simulink model "sampleModel1845"  (R2023a)
settings: Solver=VariableStepAuto  StartTime=0.0  StopTime=10.0  RelTol=1e-3
libraries: simulink x4, hdlsllib x2
settings Model: Creator=user1  LastModifiedBy=user1

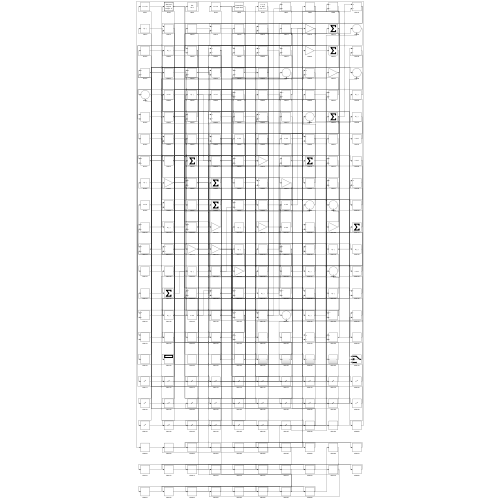
[thumbnail: Simulink's stored preview of the top-level diagram]
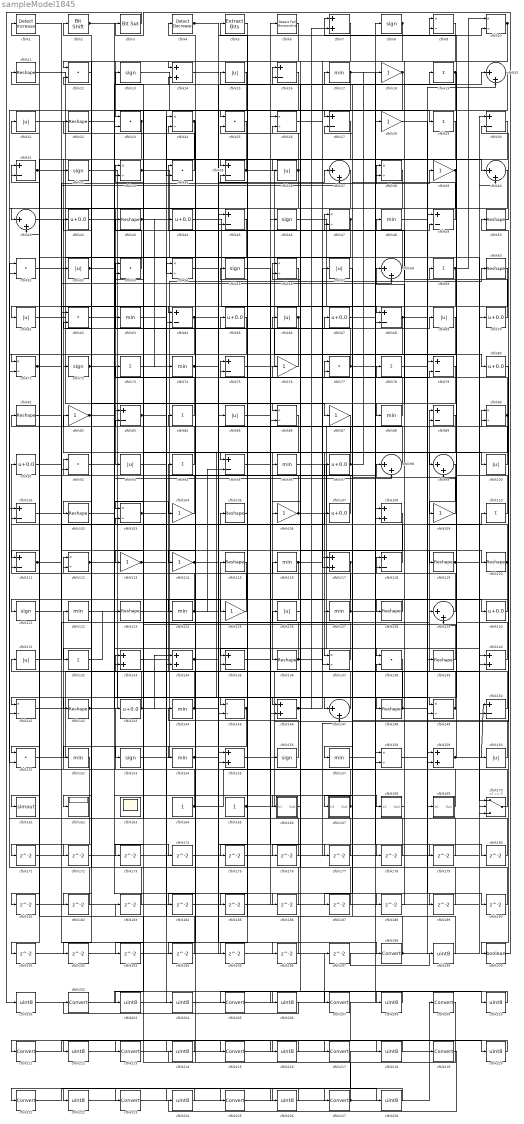
== system sampleModel1845 ==
  cfblk1 : simulink/Logic and Bit Operations/Detect Increase  vinit=0.0  OutDataTypeStr=boolean
      settings: LibrarySourceBlock=|
      | hdlsllib/Logic and Bit
      | Operations/Detect
      | Increase
  cfblk{9..10,24,26,33,38,47,54,56,71,86,90,103,112,137,141,145,149,158} (19 alike) : Product  Inputs=*/  RndMeth=Zero  SaturateOnIntegerOverflow=on
  cfblk{15,21,36,52,57,61,66,69,85,93,100,126,131,160} (14 alike) : Abs  SaturateOnIntegerOverflow=off
  cfblk{16,27,30..31,35,45,49,64,68,75,79,83,89,95,101,111,118,135,150} (19 alike) : Sum  Inputs=+-
  cfblk{11,22,43,50,60,81,102,105,115,119..120,123,128,136,139,142,148} (17 alike) : Reshape
  cfblk{18,28,39,76,82,87,104,106,109,113..114,125} (12 alike) : Gain
  cfblk{42,44,65,67,70,80,91,97,107,130,143} (11 alike) : Bias  Bias=0.0  SaturateOnIntegerOverflow=off
  cfblk{7,14,108,117,133..134,140,146,155,159} (10 alike) : Sum
  cfblk{19,29,59,73,78,84,94,110,132} (9 alike) : Sum  Inputs=+
  cfblk{17,48,63,74,88,96,116,122,124,127,144,152,154,157} (14 alike) : MinMax
  cfblk{12,23,25,34,51,53,62,77,92,138,151} (11 alike) : DotProduct  OutDataTypeStr=Inherit: Inherit via internal rule
  cfblk{8,13,32,46,55,72,121,153,156} (9 alike) : Signum
  cfblk{20,37,40..41,58,98..99,129,147} (9 alike) : Sum  Inputs=|++
  cfblk161 : ToWorkspace  VariableName=simout  SaveFormat=Timeseries  SampleTime=-1
  cfblk162 : Display
  cfblk163 : Scope
      settings: Floating=on
  cfblk164 : Constant  SampleTime=-1
  cfblk165 : Constant  SampleTime=-1
  cfblk166 : Subsystem
      settings: LibrarySourceBlock=|
      | hdlsllib/Ports &
      | Subsystems/Subsystem
  cfblk167 : Subsystem
      settings: LibrarySourceBlock=|
      | hdlsllib/Ports &
      | Subsystems/Subsystem
  cfblk168 : Subsystem
      settings: LibrarySourceBlock=|
      | hdlsllib/Ports &
      | Subsystems/Subsystem
  cfblk169 : Subsystem
      settings: LibrarySourceBlock=|
      | hdlsllib/Ports &
      | Subsystems/Subsystem
  cfblk170 : Switch  SaturateOnIntegerOverflow=off  InputSameDT=off
  cfblk{171..197} (27 alike) : Delay  SampleTime=1
  cfblk{198,202,205,207,209,211,213,215,217,219,221,223,225,227} (14 alike) : DataTypeConversion  SaturateOnIntegerOverflow=off  RndMeth=Floor
  cfblk{199,201,203..204,206,208,210,212,214,216,218,220,222,224,226,228} (16 alike) : DataTypeConversion  OutDataTypeStr=uint8  SaturateOnIntegerOverflow=off  RndMeth=Floor
  cfblk2 : hdlsllib/Logic and Bit Operations/Bit Shift  mode=Shift Left Logical  N=0
  cfblk200 : DataTypeConversion  OutDataTypeStr=boolean  SaturateOnIntegerOverflow=off  RndMeth=Floor
  cfblk3 : simulink/Logic and Bit Operations/Bit Set  iBit=0
      settings: LibrarySourceBlock=|
      | hdlsllib/Logic and Bit
      | Operations/Bit Set
  cfblk4 : simulink/Logic and Bit Operations/Detect Decrease  vinit=0.0  OutDataTypeStr=boolean
      settings: LibrarySourceBlock=|
      | hdlsllib/Logic and Bit
      | Operations/Detect
      | Decrease
  cfblk5 : simulink/Logic and Bit Operations/Extract Bits  bitsToExtract=Upper half  numBits=8  bitIdxRange=[0 7]  outScalingMode=Preserve fixed-point scaling
      settings: LibrarySourceBlock=|
      | hdlsllib/Logic and Bit
      | Operations/Extract Bits
  cfblk6 : hdlsllib/Logic and Bit Operations/Detect Fall Nonpositive  vinit=0  OutDataTypeStr=boolean
  wires:
  cfblk41/1 -> cfblk86/1
  cfblk170/1 -> cfblk122/1
  cfblk110/1 -> cfblk15/1
  cfblk148/1 -> cfblk115/1, cfblk20/2
  cfblk155/1 -> cfblk50/1
  cfblk58/1 -> cfblk34/1
  cfblk86/1 -> cfblk136/1
  cfblk104/1 -> cfblk92/1
  cfblk35/1 -> cfblk80/1, cfblk32/1
  cfblk130/1 -> cfblk128/1
  cfblk51/1 -> cfblk148/1
  cfblk64/1 -> cfblk87/1, cfblk151/2, cfblk196/1
  cfblk158/1 -> cfblk110/1
  cfblk32/1 -> cfblk145/1
  cfblk37/1 -> cfblk93/1
  cfblk94/1 -> cfblk21/1
  cfblk62/1 -> cfblk140/1
  cfblk111/1 -> cfblk31/1, cfblk37/2
  cfblk87/1 -> cfblk137/1
  cfblk125/1 -> cfblk91/1
  cfblk76/1 -> cfblk72/1
  cfblk107/1 -> cfblk81/1
  cfblk47/1 -> cfblk103/1, cfblk17/1
  cfblk102/1 -> cfblk83/1
  cfblk132/1 -> cfblk123/1
  cfblk70/1 -> cfblk47/1
  cfblk8/1 -> cfblk23/1, cfblk117/2
  cfblk133/1 -> cfblk60/1
  cfblk123/1 -> cfblk65/1
  cfblk21/1 -> cfblk54/2
  cfblk103/1 -> cfblk73/1, cfblk77/2
  cfblk144/1 -> cfblk37/1, cfblk133/2, cfblk186/1
  cfblk98/1 -> cfblk82/1
  cfblk165/1 -> cfblk70/1, cfblk35/2
  cfblk9/1 -> cfblk106/1
  cfblk44/1 -> cfblk158/1
  cfblk82/1 -> cfblk48/1, cfblk47/2
  cfblk159/1 -> cfblk150/1, cfblk99/2
  cfblk56/1 -> cfblk161/1
  cfblk22/1 -> cfblk27/1
  cfblk151/1 -> cfblk133/1
  cfblk147/1 -> cfblk94/1
  cfblk43/1 -> cfblk85/1, cfblk74/1
  cfblk139/1 -> cfblk103/2
  cfblk136/1 -> cfblk84/1, cfblk79/2
  cfblk142/1 -> cfblk6/1, cfblk78/1
  cfblk109/1 -> cfblk27/2
  cfblk153/1 -> cfblk28/1
  cfblk168/1(Out1) -> cfblk118/1
  cfblk65/1 -> cfblk71/1
  cfblk12/1 -> cfblk132/1
  cfblk77/1 -> cfblk53/1, cfblk10/2
  cfblk30/1 -> cfblk52/1
  cfblk96/1 -> cfblk170/1
  cfblk141/1 -> cfblk89/1
  cfblk105/1 -> cfblk135/1
  cfblk39/1 -> cfblk114/1, cfblk9/1
  cfblk7/1 -> cfblk14/1
  cfblk16/1 -> cfblk51/2
  cfblk97/1 -> cfblk83/2, cfblk18/1
  cfblk24/1 -> cfblk41/1, cfblk64/1
  cfblk11/1 -> cfblk160/1
  cfblk57/1 -> cfblk157/1
  cfblk114/1 -> cfblk149/2, cfblk178/1, cfblk179/1
  cfblk72/1 -> cfblk104/1, cfblk137/2
  cfblk1/1 -> cfblk198/1
  cfblk48/1 -> cfblk139/1
  cfblk90/1 -> cfblk77/1, cfblk176/1
  cfblk122/1 -> cfblk147/1
  cfblk79/1 -> cfblk102/1
  cfblk88/1 -> cfblk75/1
  cfblk92/1 -> cfblk138/1
  cfblk6/1 -> cfblk12/1
  cfblk2/1 -> cfblk188/1, cfblk189/1
  cfblk73/1 -> cfblk67/1
  cfblk66/1 -> cfblk152/1, cfblk111/1
  cfblk115/1 -> cfblk145/2
  cfblk33/1 -> cfblk140/2, cfblk36/1
  cfblk18/1 -> cfblk113/1, cfblk153/1
  cfblk134/1 -> cfblk38/1, cfblk90/2
  cfblk106/1 -> cfblk89/2, cfblk42/1
  cfblk127/1 -> cfblk63/1, cfblk130/1
  cfblk113/1 -> cfblk44/1, cfblk76/1
  cfblk150/1 -> cfblk98/1
  cfblk84/1 -> cfblk13/1
  cfblk156/1 -> cfblk24/2
  cfblk17/1 -> cfblk34/2, cfblk95/1, cfblk29/1
  cfblk145/1 -> cfblk154/1, cfblk162/1
  cfblk14/1 -> cfblk100/1
  cfblk83/1 -> cfblk96/1, cfblk125/1
  cfblk169/1(Out1) -> cfblk138/2
  cfblk15/1 -> cfblk71/2
  cfblk93/1 -> cfblk99/1
  cfblk46/1 -> cfblk158/2
  cfblk19/1 -> cfblk23/2, cfblk149/1
  cfblk129/1 -> cfblk5/1
  cfblk116/1 -> cfblk57/1, cfblk181/1
  cfblk99/1 -> cfblk109/1
  cfblk149/1 -> cfblk141/1, cfblk11/1
  cfblk135/1 -> cfblk156/1
  cfblk54/1 -> cfblk155/2
  cfblk59/1 -> cfblk167/1(In1), cfblk10/1, cfblk146/2
  cfblk26/1 -> cfblk68/1
  cfblk4/1 -> cfblk40/1, cfblk9/2
  cfblk140/1 -> cfblk7/1
  cfblk50/1 -> cfblk30/2
  cfblk91/1 -> cfblk38/2
  cfblk49/1 -> cfblk16/1
  cfblk34/1 -> cfblk2/1
  cfblk143/1 -> cfblk146/1, cfblk22/1, cfblk134/1
  cfblk25/1 -> cfblk142/1
  cfblk160/1 -> cfblk116/1
  cfblk31/1 -> cfblk45/2, cfblk64/2
  cfblk68/1 -> cfblk159/2, cfblk134/2
  cfblk126/1 -> cfblk56/1
  cfblk45/1 -> cfblk121/1
  cfblk69/1 -> cfblk92/2
  cfblk95/1 -> cfblk46/1
  cfblk146/1 -> cfblk117/1, cfblk7/2
  cfblk67/1 -> cfblk49/2
  cfblk71/1 -> cfblk120/1, cfblk58/2
  cfblk166/1(Out1) -> cfblk26/2
  cfblk119/1 -> cfblk40/2, cfblk59/1, cfblk129/2
  cfblk131/1 -> cfblk129/1
  cfblk118/1 -> cfblk56/2
  cfblk164/1 -> cfblk143/1, cfblk33/2, cfblk8/1, cfblk131/1
  cfblk137/1 -> cfblk33/1
  cfblk100/1 -> cfblk90/1
  cfblk81/1 -> cfblk119/1
  cfblk20/1 -> cfblk25/1
  cfblk55/1 -> cfblk127/1
  cfblk75/1 -> cfblk69/1
  cfblk120/1 -> cfblk101/2, cfblk75/2, cfblk175/1, cfblk187/1
  cfblk28/1 -> cfblk169/1(In1)
  cfblk154/1 -> cfblk126/1, cfblk4/1
  cfblk13/1 -> cfblk118/2
  cfblk10/1 -> cfblk88/1, cfblk182/1
  cfblk117/1 -> cfblk193/1, cfblk194/1
  cfblk101/1 -> cfblk62/1
  cfblk53/1 -> cfblk43/1
  cfblk61/1 -> cfblk66/1
  cfblk121/1 -> cfblk107/1
  cfblk74/1 -> cfblk39/1, cfblk168/1(In1)
  cfblk124/1 -> cfblk112/1, cfblk20/1, cfblk95/2
  cfblk112/1 -> cfblk166/1(In1), cfblk14/2
  cfblk36/1 -> cfblk35/1, cfblk25/2, cfblk141/2
  cfblk52/1 -> cfblk19/1, cfblk98/2
  cfblk23/1 -> cfblk61/1, cfblk151/1
  cfblk167/1(Out1) -> cfblk112/2, cfblk55/1
  cfblk128/1 -> cfblk124/1
  cfblk152/1 -> cfblk171/1
  cfblk171/1 -> cfblk147/2
  cfblk40/1 -> cfblk172/1
  cfblk172/1 -> cfblk86/2
  cfblk89/1 -> cfblk173/1
  cfblk173/1 -> cfblk49/1
  cfblk42/1 -> cfblk174/1
  cfblk174/1 -> cfblk150/2
  cfblk175/1 -> cfblk68/2
  cfblk176/1 -> cfblk135/2
  cfblk85/1 -> cfblk177/1
  cfblk177/1 -> cfblk53/2
  cfblk178/1 -> cfblk155/1
  cfblk179/1 -> cfblk62/2
  cfblk157/1 -> cfblk180/1
  cfblk180/1 -> cfblk51/1
  cfblk181/1 -> cfblk170/3
  cfblk182/1 -> cfblk31/2
  cfblk183/1 -> cfblk101/1
  cfblk27/1 -> cfblk184/1
  cfblk184/1 -> cfblk30/1
  cfblk60/1 -> cfblk185/1
  cfblk185/1 -> cfblk26/1
  cfblk186/1 -> cfblk12/2
  cfblk187/1 -> cfblk16/2
  cfblk188/1 -> cfblk58/1
  cfblk189/1 -> cfblk111/2
  cfblk78/1 -> cfblk190/1
  cfblk190/1 -> cfblk24/1
  cfblk29/1 -> cfblk191/1
  cfblk191/1 -> cfblk159/1
  cfblk38/1 -> cfblk192/1
  cfblk192/1 -> cfblk45/1
  cfblk193/1 -> cfblk170/2
  cfblk194/1 -> cfblk41/2
  cfblk5/1 -> cfblk195/1
  cfblk195/1 -> cfblk79/1
  cfblk196/1 -> cfblk54/1
  cfblk198/1 -> cfblk97/1, cfblk105/1
  cfblk197/1 -> cfblk199/1
  cfblk199/1 -> cfblk1/1
  cfblk80/1 -> cfblk200/1
  cfblk200/1 -> cfblk3/1
  cfblk3/1 -> cfblk201/1
  cfblk201/1 -> cfblk197/1
  cfblk138/1 -> cfblk203/1
  cfblk203/1 -> cfblk108/1
  cfblk63/1 -> cfblk204/1
  cfblk204/1 -> cfblk108/2
  cfblk108/1 -> cfblk206/1
  cfblk206/1 -> cfblk202/1
  cfblk202/1 -> cfblk208/1
  cfblk208/1 -> cfblk205/1
  cfblk205/1 -> cfblk210/1
  cfblk210/1 -> cfblk207/1
  cfblk207/1 -> cfblk212/1
  cfblk212/1 -> cfblk209/1
  cfblk209/1 -> cfblk214/1
  cfblk214/1 -> cfblk211/1
  cfblk211/1 -> cfblk216/1
  cfblk216/1 -> cfblk213/1
  cfblk213/1 -> cfblk218/1
  cfblk218/1 -> cfblk215/1
  cfblk215/1 -> cfblk220/1
  cfblk220/1 -> cfblk217/1
  cfblk217/1 -> cfblk222/1
  cfblk222/1 -> cfblk219/1
  cfblk219/1 -> cfblk224/1
  cfblk224/1 -> cfblk221/1
  cfblk225/1 -> cfblk227/1
  cfblk221/1 -> cfblk226/1
  cfblk226/1 -> cfblk223/1
  cfblk227/1 -> cfblk183/1, cfblk144/1
  cfblk223/1 -> cfblk228/1
  cfblk228/1 -> cfblk225/1

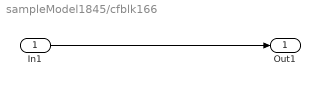
== system sampleModel1845/cfblk166 ==
  In1 : Inport
  Out1 : Outport
  wires:
  In1/1 -> Out1/1

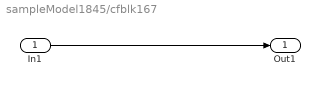
== system sampleModel1845/cfblk167 ==
  In1 : Inport
  Out1 : Outport
  wires:
  In1/1 -> Out1/1

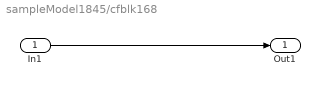
== system sampleModel1845/cfblk168 ==
  In1 : Inport
  Out1 : Outport
  wires:
  In1/1 -> Out1/1

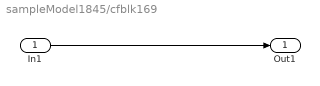
== system sampleModel1845/cfblk169 ==
  In1 : Inport
  Out1 : Outport
  wires:
  In1/1 -> Out1/1
